simulink model "hw3_sim"  (R2022a)
settings: Solver=VariableStepAuto  StartTime=0.0  StopTime=20  RelTol=1e-3
values from neighbouring files (symbols this model uses):
  A = [ ... (first row only)    [hw3.m]    (also in maglev.m = raw_A - B*K_leader)
  Adj = full(adjacency(Gr))    [hw3.m]    (also in maglev.m = full(adjacency(Gr, 'weighted')))
  B = [0; 1/m1; 0; 0]    [hw3.m]    (also in maglev.m = [0; -9.9453])
  c = 0.7    [hw3.m]    (also in maglev.m = c_values(i))
  C = eye(4)    [hw3.m]    (also in maglev.m = [708.27 0])
  K = inv(R)*(B')*P    [hw3.m]    (also in maglev.m)
  pins = [1 0 0 0 0 0]    [hw3.m]    (also in maglev.m)
settings Model: Creator=jules  LastModifiedBy=jules
settings DebuggingCC: AllowedUnitSystems=SI,SI (extended)

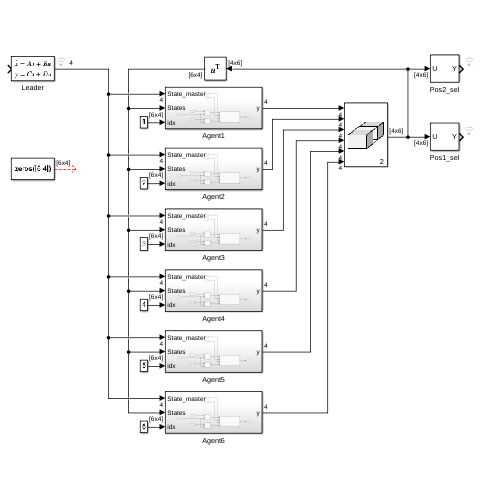
[thumbnail: Simulink's stored preview of the top-level diagram]
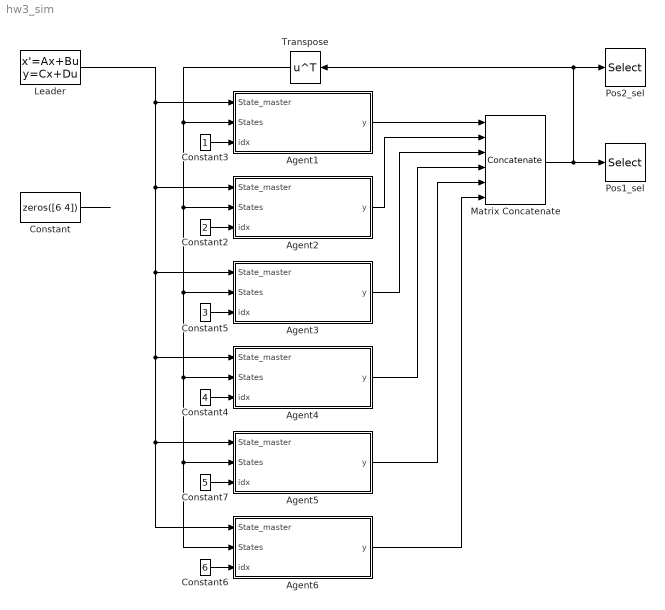
== system hw3_sim ==
  Agent1 : Subsystem
  Agent2 : Subsystem
  Agent3 : Subsystem
  Agent4 : Subsystem
  Agent5 : Subsystem
  Agent6 : Subsystem
  Constant : Constant  Value=zeros([6 4])
  Constant2 : Constant  Value=2
  Constant3 : Constant
  Constant4 : Constant  Value=4
  Constant5 : Constant  Value=3
  Constant6 : Constant  Value=6
  Constant7 : Constant  Value=5
  Leader : StateSpace  A=A  B=zeros([4 1])  C=C  D=zeros([4 1])  InitialCondition=[10 0 0 0]
  Matrix Concatenate : Concatenate  NumInputs=6  Mode=Multidimensional array  ConcatenateDimension=2
  Pos1_sel : Selector  NumberOfDimensions=2  InputPortWidth=3  IndexOptions=Index vector (dialog),Select all  Indices=1,1  OutputSizes=1,1
  Pos2_sel : Selector  NumberOfDimensions=2  InputPortWidth=3  IndexOptions=Index vector (dialog),Select all  Indices=1,3  OutputSizes=1,1
  Transpose : Math  Operator=transpose
  wires:
  Leader/1 -> Agent1/1(State_master), Agent2/1(State_master), Agent3/1(State_master), Agent4/1(State_master), Agent5/1(State_master), Agent6/1(State_master)
  Constant3/1 -> Agent1/3(idx)
  Constant2/1 -> Agent2/3(idx)
  Constant4/1 -> Agent4/3(idx)
  Constant5/1 -> Agent3/3(idx)
  Constant6/1 -> Agent6/3(idx)
  Constant7/1 -> Agent5/3(idx)
  Agent1/1(y) -> Matrix Concatenate/1
  Agent2/1(y) -> Matrix Concatenate/2
  Matrix Concatenate/1 -> Transpose/1, Pos2_sel/1, Pos1_sel/1
  Agent3/1(y) -> Matrix Concatenate/3
  Agent4/1(y) -> Matrix Concatenate/4
  Agent5/1(y) -> Matrix Concatenate/5
  Agent6/1(y) -> Matrix Concatenate/6
  Constant/1 -> ?
  Transpose/1 -> Agent2/2(States), Agent3/2(States), Agent4/2(States), Agent5/2(States), Agent6/2(States), Agent1/2(States)

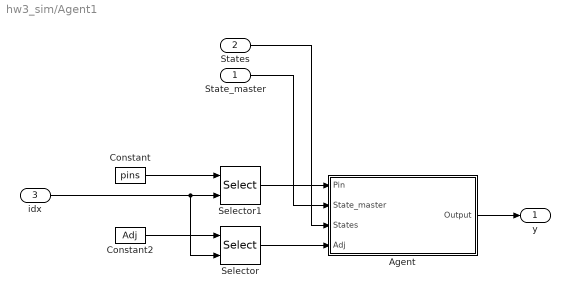
== system hw3_sim/Agent1 ==
  State_master : Inport
  States : Inport  Port=2
  idx : Inport  Port=3
  Agent : Subsystem
  Constant : Constant  Value=pins
  Constant2 : Constant  Value=Adj  VectorParams1D=off
  Selector : Selector  NumberOfDimensions=2  InputPortWidth=[6 6]  IndexOptions=Select all,Index vector (port)  Indices=[1 3],1  OutputSizes=1,1
  Selector1 : Selector  InputPortWidth=6  IndexOptions=Index vector (port)  Indices=[1 3]  OutputSizes=1
  y : Outport
  wires:
  Selector1/1 -> Agent/1(Pin)
  idx/1 -> Selector1/2, Selector/2
  Selector/1 -> Agent/4(Adj)
  Constant2/1 -> Selector/1
  Agent/1(Output) -> y/1
  Constant/1 -> Selector1/1
  States/1 -> Agent/3(States)
  State_master/1 -> Agent/2(State_master)

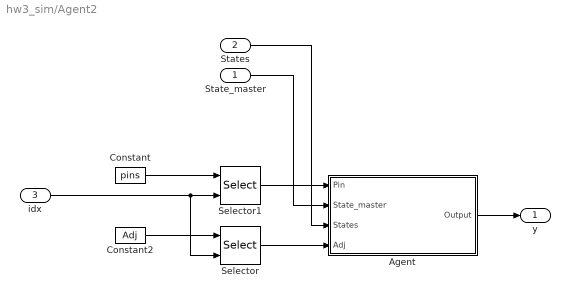
== system hw3_sim/Agent2 ==
  State_master : Inport
  States : Inport  Port=2
  idx : Inport  Port=3
  Agent : Subsystem
  Constant : Constant  Value=pins
  Constant2 : Constant  Value=Adj  VectorParams1D=off
  Selector : Selector  NumberOfDimensions=2  InputPortWidth=[6 6]  IndexOptions=Select all,Index vector (port)  Indices=[1 3],1  OutputSizes=1,1
  Selector1 : Selector  InputPortWidth=6  IndexOptions=Index vector (port)  Indices=[1 3]  OutputSizes=1
  y : Outport
  wires:
  Selector1/1 -> Agent/1(Pin)
  idx/1 -> Selector1/2, Selector/2
  Selector/1 -> Agent/4(Adj)
  Constant2/1 -> Selector/1
  Agent/1(Output) -> y/1
  Constant/1 -> Selector1/1
  States/1 -> Agent/3(States)
  State_master/1 -> Agent/2(State_master)

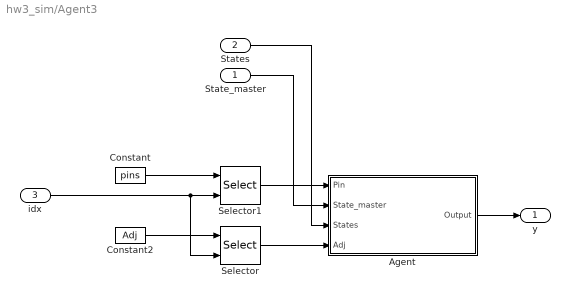
== system hw3_sim/Agent3 ==
  State_master : Inport
  States : Inport  Port=2
  idx : Inport  Port=3
  Agent : Subsystem
  Constant : Constant  Value=pins
  Constant2 : Constant  Value=Adj  VectorParams1D=off
  Selector : Selector  NumberOfDimensions=2  InputPortWidth=[6 6]  IndexOptions=Select all,Index vector (port)  Indices=[1 3],1  OutputSizes=1,1
  Selector1 : Selector  InputPortWidth=6  IndexOptions=Index vector (port)  Indices=[1 3]  OutputSizes=1
  y : Outport
  wires:
  Selector1/1 -> Agent/1(Pin)
  idx/1 -> Selector1/2, Selector/2
  Selector/1 -> Agent/4(Adj)
  Constant2/1 -> Selector/1
  Agent/1(Output) -> y/1
  Constant/1 -> Selector1/1
  States/1 -> Agent/3(States)
  State_master/1 -> Agent/2(State_master)

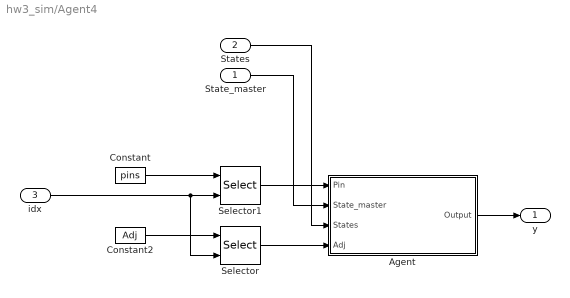
== system hw3_sim/Agent4 ==
  State_master : Inport
  States : Inport  Port=2
  idx : Inport  Port=3
  Agent : Subsystem
  Constant : Constant  Value=pins
  Constant2 : Constant  Value=Adj  VectorParams1D=off
  Selector : Selector  NumberOfDimensions=2  InputPortWidth=[6 6]  IndexOptions=Select all,Index vector (port)  Indices=[1 3],1  OutputSizes=1,1
  Selector1 : Selector  InputPortWidth=6  IndexOptions=Index vector (port)  Indices=[1 3]  OutputSizes=1
  y : Outport
  wires:
  Selector1/1 -> Agent/1(Pin)
  idx/1 -> Selector1/2, Selector/2
  Selector/1 -> Agent/4(Adj)
  Constant2/1 -> Selector/1
  Agent/1(Output) -> y/1
  Constant/1 -> Selector1/1
  States/1 -> Agent/3(States)
  State_master/1 -> Agent/2(State_master)

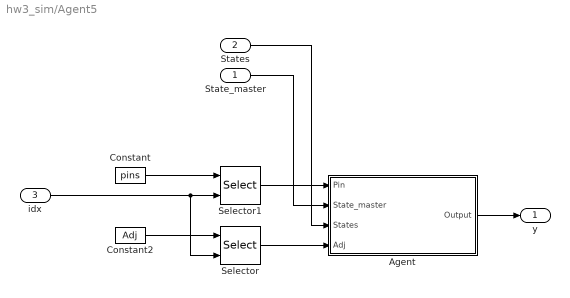
== system hw3_sim/Agent5 ==
  State_master : Inport
  States : Inport  Port=2
  idx : Inport  Port=3
  Agent : Subsystem
  Constant : Constant  Value=pins
  Constant2 : Constant  Value=Adj  VectorParams1D=off
  Selector : Selector  NumberOfDimensions=2  InputPortWidth=[6 6]  IndexOptions=Select all,Index vector (port)  Indices=[1 3],1  OutputSizes=1,1
  Selector1 : Selector  InputPortWidth=6  IndexOptions=Index vector (port)  Indices=[1 3]  OutputSizes=1
  y : Outport
  wires:
  Selector1/1 -> Agent/1(Pin)
  idx/1 -> Selector1/2, Selector/2
  Selector/1 -> Agent/4(Adj)
  Constant2/1 -> Selector/1
  Agent/1(Output) -> y/1
  Constant/1 -> Selector1/1
  States/1 -> Agent/3(States)
  State_master/1 -> Agent/2(State_master)

== system hw3_sim/Agent6 ==
  State_master : Inport
  States : Inport  Port=2
  idx : Inport  Port=3
  Agent : Subsystem
  Constant : Constant  Value=pins
  Constant2 : Constant  Value=Adj  VectorParams1D=off
  Selector : Selector  NumberOfDimensions=2  InputPortWidth=[6 6]  IndexOptions=Select all,Index vector (port)  Indices=[1 3],1  OutputSizes=1,1
  Selector1 : Selector  InputPortWidth=6  IndexOptions=Index vector (port)  Indices=[1 3]  OutputSizes=1
  y : Outport
  wires:
  Selector1/1 -> Agent/1(Pin)
  idx/1 -> Selector1/2, Selector/2
  Selector/1 -> Agent/4(Adj)
  Constant2/1 -> Selector/1
  Agent/1(Output) -> y/1
  Constant/1 -> Selector1/1
  States/1 -> Agent/3(States)
  State_master/1 -> Agent/2(State_master)

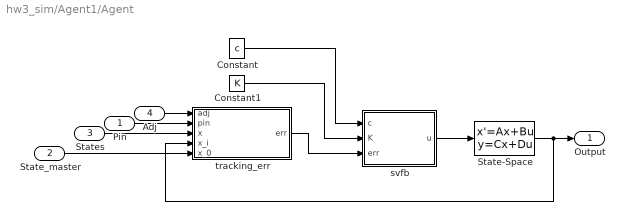
== system hw3_sim/Agent1/Agent ==
  Pin : Inport
  State_master : Inport  Port=2  PortDimensions=4
  States : Inport  Port=3
  Adj : Inport  Port=4  PortDimensions=6
  Constant : Constant  Value=c
  Constant1 : Constant  Value=K  VectorParams1D=off
  State-Space : StateSpace  A=A  B=B  C=C  D=zeros([4 1])  InitialCondition=0
  svfb : MATLAB Function  TreatAsAtomicUnit=on
  tracking_err : MATLAB Function  TreatAsAtomicUnit=on
  Output : Outport
  wires:
  Adj/1 -> tracking_err/1(adj)
  Pin/1 -> tracking_err/2(pin)
  State_master/1 -> tracking_err/5(x_0)
  States/1 -> tracking_err/3(x)
  Constant/1 -> svfb/1(c)
  Constant1/1 -> svfb/2(K)
  tracking_err/1(err) -> svfb/3(err)
  State-Space/1 -> tracking_err/4(x_i), Output/1
  svfb/1(u) -> State-Space/1

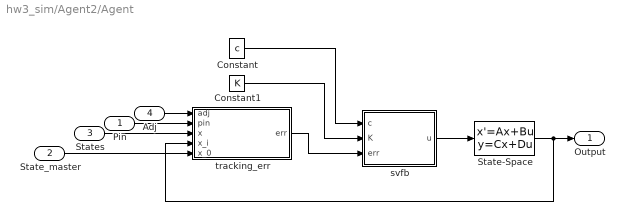
== system hw3_sim/Agent2/Agent ==
  Pin : Inport
  State_master : Inport  Port=2  PortDimensions=4
  States : Inport  Port=3
  Adj : Inport  Port=4  PortDimensions=6
  Constant : Constant  Value=c
  Constant1 : Constant  Value=K  VectorParams1D=off
  State-Space : StateSpace  A=A  B=B  C=C  D=zeros([4 1])  InitialCondition=0
  svfb : MATLAB Function  TreatAsAtomicUnit=on
  tracking_err : MATLAB Function  TreatAsAtomicUnit=on
  Output : Outport
  wires:
  Adj/1 -> tracking_err/1(adj)
  Pin/1 -> tracking_err/2(pin)
  State_master/1 -> tracking_err/5(x_0)
  States/1 -> tracking_err/3(x)
  Constant/1 -> svfb/1(c)
  Constant1/1 -> svfb/2(K)
  tracking_err/1(err) -> svfb/3(err)
  State-Space/1 -> tracking_err/4(x_i), Output/1
  svfb/1(u) -> State-Space/1

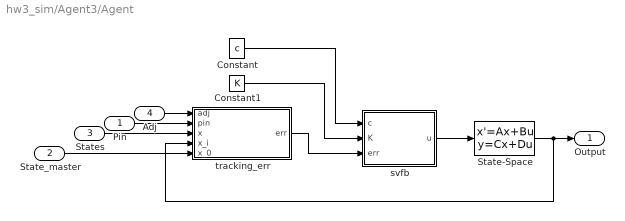
== system hw3_sim/Agent3/Agent ==
  Pin : Inport
  State_master : Inport  Port=2  PortDimensions=4
  States : Inport  Port=3
  Adj : Inport  Port=4  PortDimensions=6
  Constant : Constant  Value=c
  Constant1 : Constant  Value=K  VectorParams1D=off
  State-Space : StateSpace  A=A  B=B  C=C  D=zeros([4 1])  InitialCondition=0
  svfb : MATLAB Function  TreatAsAtomicUnit=on
  tracking_err : MATLAB Function  TreatAsAtomicUnit=on
  Output : Outport
  wires:
  Adj/1 -> tracking_err/1(adj)
  Pin/1 -> tracking_err/2(pin)
  State_master/1 -> tracking_err/5(x_0)
  States/1 -> tracking_err/3(x)
  Constant/1 -> svfb/1(c)
  Constant1/1 -> svfb/2(K)
  tracking_err/1(err) -> svfb/3(err)
  State-Space/1 -> tracking_err/4(x_i), Output/1
  svfb/1(u) -> State-Space/1

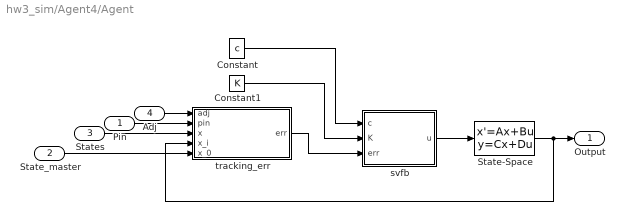
== system hw3_sim/Agent4/Agent ==
  Pin : Inport
  State_master : Inport  Port=2  PortDimensions=4
  States : Inport  Port=3
  Adj : Inport  Port=4  PortDimensions=6
  Constant : Constant  Value=c
  Constant1 : Constant  Value=K  VectorParams1D=off
  State-Space : StateSpace  A=A  B=B  C=C  D=zeros([4 1])  InitialCondition=0
  svfb : MATLAB Function  TreatAsAtomicUnit=on
  tracking_err : MATLAB Function  TreatAsAtomicUnit=on
  Output : Outport
  wires:
  Adj/1 -> tracking_err/1(adj)
  Pin/1 -> tracking_err/2(pin)
  State_master/1 -> tracking_err/5(x_0)
  States/1 -> tracking_err/3(x)
  Constant/1 -> svfb/1(c)
  Constant1/1 -> svfb/2(K)
  tracking_err/1(err) -> svfb/3(err)
  State-Space/1 -> tracking_err/4(x_i), Output/1
  svfb/1(u) -> State-Space/1

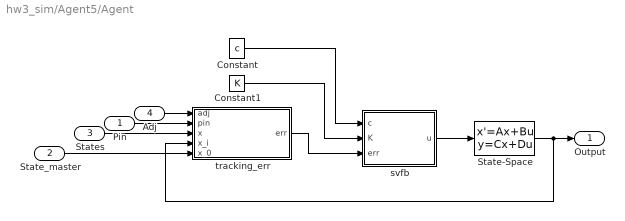
== system hw3_sim/Agent5/Agent ==
  Pin : Inport
  State_master : Inport  Port=2  PortDimensions=4
  States : Inport  Port=3
  Adj : Inport  Port=4  PortDimensions=6
  Constant : Constant  Value=c
  Constant1 : Constant  Value=K  VectorParams1D=off
  State-Space : StateSpace  A=A  B=B  C=C  D=zeros([4 1])  InitialCondition=0
  svfb : MATLAB Function  TreatAsAtomicUnit=on
  tracking_err : MATLAB Function  TreatAsAtomicUnit=on
  Output : Outport
  wires:
  Adj/1 -> tracking_err/1(adj)
  Pin/1 -> tracking_err/2(pin)
  State_master/1 -> tracking_err/5(x_0)
  States/1 -> tracking_err/3(x)
  Constant/1 -> svfb/1(c)
  Constant1/1 -> svfb/2(K)
  tracking_err/1(err) -> svfb/3(err)
  State-Space/1 -> tracking_err/4(x_i), Output/1
  svfb/1(u) -> State-Space/1

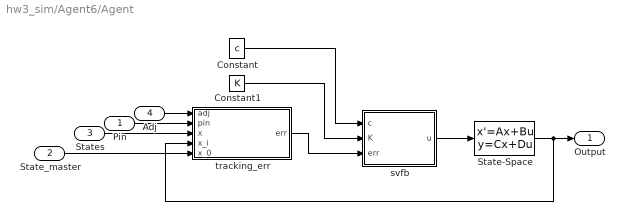
== system hw3_sim/Agent6/Agent ==
  Pin : Inport
  State_master : Inport  Port=2  PortDimensions=4
  States : Inport  Port=3
  Adj : Inport  Port=4  PortDimensions=6
  Constant : Constant  Value=c
  Constant1 : Constant  Value=K  VectorParams1D=off
  State-Space : StateSpace  A=A  B=B  C=C  D=zeros([4 1])  InitialCondition=0
  svfb : MATLAB Function  TreatAsAtomicUnit=on
  tracking_err : MATLAB Function  TreatAsAtomicUnit=on
  Output : Outport
  wires:
  Adj/1 -> tracking_err/1(adj)
  Pin/1 -> tracking_err/2(pin)
  State_master/1 -> tracking_err/5(x_0)
  States/1 -> tracking_err/3(x)
  Constant/1 -> svfb/1(c)
  Constant1/1 -> svfb/2(K)
  tracking_err/1(err) -> svfb/3(err)
  State-Space/1 -> tracking_err/4(x_i), Output/1
  svfb/1(u) -> State-Space/1

== matlab function hw3_sim/Agent5/Agent/tracking_err ==
  data: adj input; pin input; x input; x_i input; x_0 input; err output
function err = tracking_err(adj, pin, x, x_i, x_0)
err = zeros([4 1]);
err = err + pin * (x_0 - x_i);
for j = 1:6
    err = err + adj(j) * (x(j) - x_i);
end

== matlab function hw3_sim/Agent6/Agent/svfb ==
  data: c input; K input; u output; err input
function u = svfb(c, K, err)
u = 0;
u = u + (c * K * err)';

== matlab function hw3_sim/Agent1/Agent/svfb ==
  data: c input; K input; u output; err input
function u = svfb(c, K, err)
u = 0;
u = u + (c * K * err)';

== matlab function hw3_sim/Agent6/Agent/tracking_err ==
  data: adj input; pin input; x input; x_i input; x_0 input; err output
function err = tracking_err(adj, pin, x, x_i, x_0)
err = zeros([4 1]);
err = err + pin * (x_0 - x_i);
for j = 1:6
    err = err + adj(j) * (x(j) - x_i);
end

== matlab function hw3_sim/Agent1/Agent/tracking_err ==
  data: adj input; pin input; x input; x_i input; x_0 input; err output
function err = tracking_err(adj, pin, x, x_i, x_0)
err = zeros([4 1]);
err = err + pin * (x_0 - x_i);
for j = 1:6
    err = err + adj(j) * (x(j) - x_i);
end

== matlab function hw3_sim/Agent2/Agent/svfb ==
  data: c input; K input; u output; err input
function u = svfb(c, K, err)
u = 0;
u = u + (c * K * err)';

== matlab function hw3_sim/Agent2/Agent/tracking_err ==
  data: adj input; pin input; x input; x_i input; x_0 input; err output
function err = tracking_err(adj, pin, x, x_i, x_0)
err = zeros([4 1]);
err = err + pin * (x_0 - x_i);
for j = 1:6
    err = err + adj(j) * (x(j) - x_i);
end

== matlab function hw3_sim/Agent3/Agent/svfb ==
  data: c input; K input; u output; err input
function u = svfb(c, K, err)
u = 0;
u = u + (c * K * err)';

== matlab function hw3_sim/Agent3/Agent/tracking_err ==
  data: adj input; pin input; x input; x_i input; x_0 input; err output
function err = tracking_err(adj, pin, x, x_i, x_0)
err = zeros([4 1]);
err = err + pin * (x_0 - x_i);
for j = 1:6
    err = err + adj(j) * (x(j) - x_i);
end

== matlab function hw3_sim/Agent4/Agent/svfb ==
  data: c input; K input; u output; err input
function u = svfb(c, K, err)
u = 0;
u = u + (c * K * err)';

== matlab function hw3_sim/Agent4/Agent/tracking_err ==
  data: adj input; pin input; x input; x_i input; x_0 input; err output
function err = tracking_err(adj, pin, x, x_i, x_0)
err = zeros([4 1]);
err = err + pin * (x_0 - x_i);
for j = 1:6
    err = err + adj(j) * (x(j) - x_i);
end

== matlab function hw3_sim/Agent5/Agent/svfb ==
  data: c input; K input; u output; err input
function u = svfb(c, K, err)
u = 0;
u = u + (c * K * err)';
